simulink model "PV_microgrid"  (R2022b)
settings: Solver=FixedStepAuto  StartTime=0.0  StopTime=0.6  FixedStep=1e-6  RelTol=1e-3
model workspace (MAT data in the model file):
  C = 0.002
  D = 100
  GP = 1
  GQ = 1
  I1 = 100
  I2 = 50
  J = 3.5
  KQ = 0.06
  Kf = 120
  Kv = 577
  L = 2e-05
  LS = 0.003
  P1 = 0.2
  P2 = 6
  Pref = 500000
  Qref = 0
  Ts = 0.0001
  Ts_power = 1e-06
  Ug = 563.38264084
  fsw = 10000
  t0 = 0.5
  wn = 314.159265359
undefined symbols (not defined in the file): D1, Delta, DiscIntNeverNeededParam, Ion, Lithium, LL, LP, Ts_Power
libraries: spsSeriesRLCBranchLib x9, spsFirstOrderFilterLib x7, slpidlib x5, spsMeanLib x5, spsabctodq0Lib x4, spsStairGeneratorLib x4, spsThreePhaseVIMeasurementLib x3, spsThreePhaseTransformerTwoWindingsLib x2, spsThreePhaseParallelRLCLoadLib x2, spsThreePhasePISectionLineLib x2, spsBoostConverterLib x2, spsPowerPositiveSequenceLib x2
(part 2 of 2)

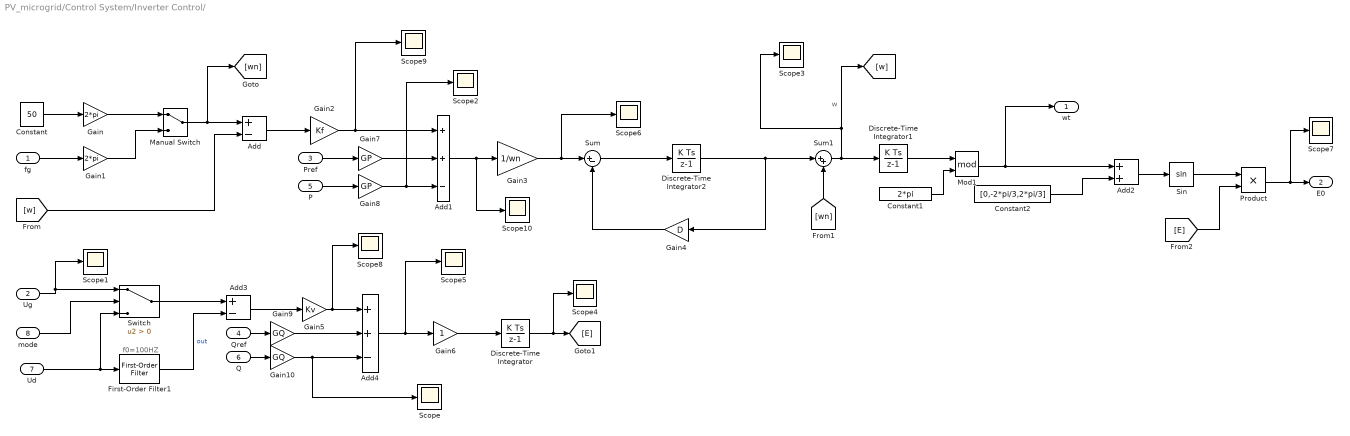
== system PV_microgrid/Control System/Inverter Control/   ==
  note: f0=100HZ
  note: w
  fg : Inport
  Ug : Inport  Port=2
  Pref : Inport  Port=3
  Qref : Inport  Port=4
  P : Inport  Port=5
  Q : Inport  Port=6
  Ud : Inport  Port=7
  mode : Inport  Port=8
  Add : Sum  Inputs=+-
  Add1 : Sum  Inputs=++-
  Add2 : Sum
  Add3 : Sum  Inputs=+-
  Add4 : Sum  Inputs=++-
  Constant : Constant  Value=50
  Constant1 : Constant  Value=2*pi
  Constant2 : Constant  Value=[0,-2*pi/3,2*pi/3]
  Discrete-Time Integrator : DiscreteIntegrator  gainval=KQ  SampleTime=1/fsw  ICPrevOutput=DiscIntNeverNeededParam  ICPrevScaledInput=DiscIntNeverNeededParam
  Discrete-Time Integrator1 : DiscreteIntegrator  SampleTime=1/fsw  ICPrevOutput=DiscIntNeverNeededParam  ICPrevScaledInput=DiscIntNeverNeededParam
  Discrete-Time Integrator2 : DiscreteIntegrator  gainval=1/J  SampleTime=1/fsw  ICPrevOutput=DiscIntNeverNeededParam  ICPrevScaledInput=DiscIntNeverNeededParam
  First-Order Filter1 : spsFirstOrderFilterLib/First-Order Filter  FilterType=Lowpass  Tc=10e-3  Ts=1/fsw  Initialize=on  Vac_Init=[0, 0, 10]  Vdc_Init=0  PlotResponse=off  FreqRange="[0,  200,  1]"
  Gain : Gain  Gain=2*pi
  Gain1 : Gain  Gain=2*pi
  Gain10 : Gain  Gain=GQ
  Gain2 : Gain  Gain=Kf
  Gain3 : Gain  Gain=1/wn
  Gain4 : Gain  Gain=D
  Gain5 : Gain  Gain=Kv
  Gain6 : Gain
  Gain7 : Gain  Gain=GP
  Gain8 : Gain  Gain=GP
  Gain9 : Gain  Gain=GQ
  Manual Switch : ManualSwitch
  Mod1 : Math  Operator=mod
  Product : Product
  Scope{,1..10} (11 alike) : Scope
  Sin : Trigonometry
  Sum : Sum  Inputs=|+-
  Sum1 : Sum  Inputs=|++
  Switch : Switch  Criteria=u2 > Threshold  SaturateOnIntegerOverflow=off  InputSameDT=off
  wt : Outport
  E0 : Outport  Port=2
  wires:
  Ug/1 -> Switch/1, Scope1/1
  Gain3/1 -> Scope6/1, Sum/1
  Gain2/1 -> Scope9/1, Add1/1
  Product/1 -> Scope7/1, E0/1
  Add/1 -> Gain2/1
  [E] -> Product/2
  Add4/1 -> Scope5/1, Gain6/1
  Mod1/1 -> wt/1, Add2/1
  Sum1/1 -> Discrete-Time Integrator1/1, Scope3/1, [w]
  fg/1 -> Gain1/1
  Constant2/1 -> Add2/2
  First-Order Filter1/1 -> Add3/2  "out"
  Ud/1 -> Switch/3, First-Order Filter1/1
  Constant/1 -> Gain/1
  Sin/1 -> Product/1
  Add2/1 -> Sin/1
  Gain4/1 -> Sum/2
  P/1 -> Gain8/1
  Gain/1 -> Manual Switch/1
  Gain1/1 -> Manual Switch/2
  Discrete-Time Integrator2/1 -> Gain4/1, Sum1/1
  Constant1/1 -> Mod1/2
  Gain5/1 -> Scope8/1, Add4/1
  Q/1 -> Gain10/1
  Manual Switch/1 -> [wn], Add/1
  Pref/1 -> Gain7/1
  Add1/1 -> Scope10/1, Gain3/1
  Add3/1 -> Gain5/1
  Gain6/1 -> Discrete-Time Integrator/1
  Qref/1 -> Gain9/1
  [wn] -> Sum1/2
  Sum/1 -> Discrete-Time Integrator2/1
  Discrete-Time Integrator/1 -> Scope4/1, [E]
  Discrete-Time Integrator1/1 -> Mod1/1
  [w] -> Add/2
  Gain7/1 -> Add1/2
  Gain8/1 -> Scope2/1, Add1/3
  Gain9/1 -> Add4/2
  Gain10/1 -> Scope/1, Add4/3
  Switch/1 -> Add3/1
  mode/1 -> Switch/2

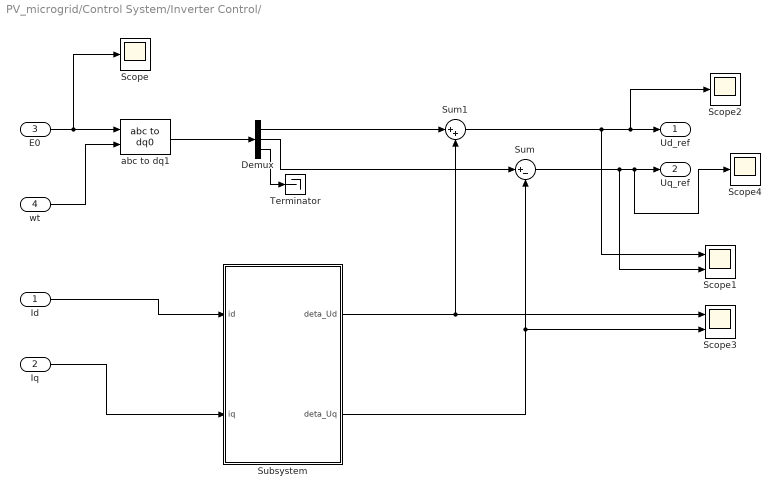
== system PV_microgrid/Control System/Inverter Control/    ==
  Id : Inport
  Iq : Inport  Port=2
  E0 : Inport  Description=Cont  Port=3
  wt : Inport  Port=4
  Demux : Demux  Outputs=3
  Scope : Scope
  Scope1 : Scope  NumInputPorts=2
  Scope2 : Scope
  Scope3 : Scope  NumInputPorts=2
  Scope4 : Scope
  Subsystem : Subsystem
  Sum : Sum  Inputs=|+-
  Sum1 : Sum  Inputs=|++
  Terminator : Terminator
  abc to dq1 : spsabctodq0Lib/abc to dq0  Alignment=90 degrees behind phase A axis
  Ud_ref : Outport
  Uq_ref : Outport  Port=2
  wires:
  Demux/1 -> Sum1/1
  E0/1 -> Scope/1, abc to dq1/1
  Id/1 -> Subsystem/1(id)
  abc to dq1/1 -> Demux/1
  Subsystem/2(deta_Uq) -> Scope3/2, Sum/2
  Sum1/1 -> Scope2/1, Ud_ref/1, Scope1/1
  wt/1 -> abc to dq1/2
  Demux/2 -> Sum/1
  Subsystem/1(deta_Ud) -> Sum1/2, Scope3/1
  Iq/1 -> Subsystem/2(iq)
  Sum/1 -> Scope4/1, Uq_ref/1, Scope1/2
  Demux/3 -> Terminator/1

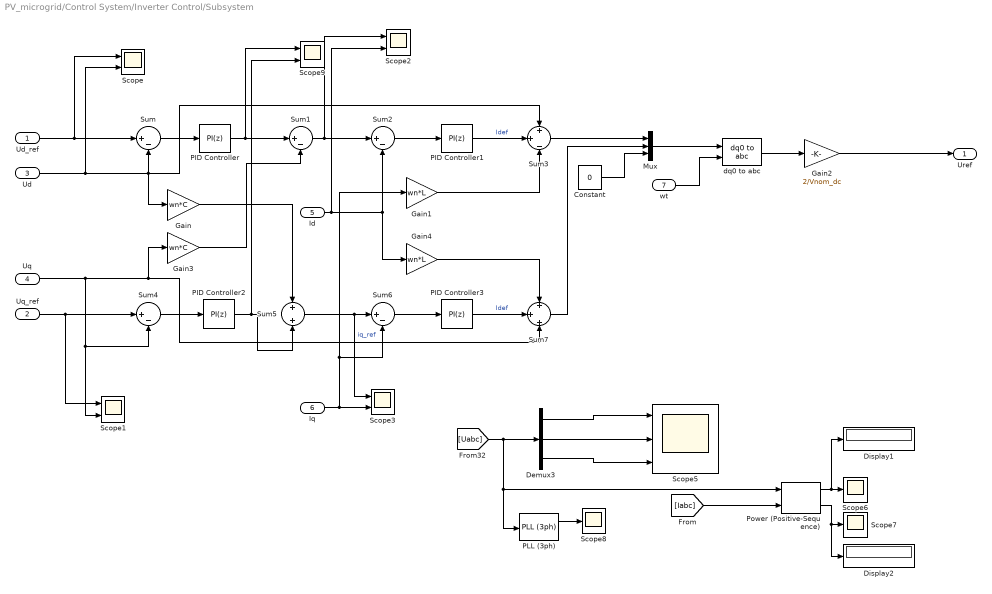
== system PV_microgrid/Control System/Inverter Control/Subsystem ==
  Ud_ref : Inport
  Uq_ref : Inport  Port=2
  Ud : Inport  Port=3
  Uq : Inport  Port=4
  Id : Inport  Port=5
  Iq : Inport  Port=6
  wt : Inport  Port=7
  Constant : Constant  Value=0
  Demux3 : Demux  Outputs=3
  Display1 : Display
  Display2 : Display
  Gain : Gain  Gain=wn*C
  Gain1 : Gain  Gain=wn*L
  Gain2 : Gain  Gain=2/Vnom_dc
  Gain3 : Gain  Gain=wn*C
  Gain4 : Gain  Gain=wn*L
  Mux : Mux  Inputs=3
  PID Controller : slpidlib/PID Controller  Controller=PI  Form=Parallel  TimeDomain=Discrete-time  UseExternalTs=off  SampleTime=-1  IntegratorMethod=Forward Euler  FilterMethod=Forward Euler  ControllerParametersSource=internal  P=P1  I=I1  UseKiTs=off  D=0  N=100  UseFilter=on  TunerSelectOption=Transfer Function Based (PID Tuner App)  InitialConditionSource=internal  InitialConditionForIntegrator=0  InitialConditionForFilter=0  DifferentiatorICPrevScaledInput=0  ExternalReset=none  TrackingMode=off  Kt=1  LimitOutput=off  SatLimitsSource=internal  UpperSaturationLimit=LP  LowerSaturationLimit=LL  LinearizeAsGain=on  AntiWindupMode=none  Kb=1  LimitIntegrator=off  UpperIntegratorSaturationLimit=inf  LowerIntegratorSaturationLimit=-inf  POutMin=[]  POutMax=[]  IOutMin=[]  IOutMax=[]  DOutMin=[]  DOutMax=[]  NOutMin=[]  NOutMax=[]  SumOutMin=[]  SumOutMax=[]  SaturationOutMin=[]  SaturationOutMax=[]  PParamMin=[]  PParamMax=[]  IParamMin=[]  IParamMax=[]  DParamMin=[]  DParamMax=[]  NParamMin=[]  NParamMax=[]  KbParamMin=[]  KbParamMax=[]  KtParamMin=[]  KtParamMax=[]  KbOutMin=[]  KbOutMax=[]  KtOutMin=[]  KtOutMax=[]  IntegratorOutMin=[]  IntegratorOutMax=[]  FilterOutMin=[]  FilterOutMax=[]  SumI1OutMin=[]  SumI1OutMax=[]  SumI2OutMin=[]  SumI2OutMax=[]  SumI3OutMin=[]  SumI3OutMax=[]  SumI4OutMin=[]  SumI4OutMax=[]  SumDOutMin=[]  SumDOutMax=[]  DifferentiatorOutMin=[]  DifferentiatorOutMax=[]  FilterDiffOutCoefMin=[]  FilterDiffOutCoefMax=[]  ReciprocalOutMin=[]  ReciprocalOutMax=[]  SumDenOutMin=[]  SumDenOutMax=[]  SumNumOutMin=[]  SumNumOutMax=[]  DivideOutMin=[]  DivideOutMax=[]  UdiffTsProdOutMin=[]  UdiffTsProdOutMax=[]  NTsProdOutMin=[]  NTsProdOutMax=[]  UintegralTsProdOutMin=[]  UintegralTsProdOutMax=[]  UngainTsProdOutMin=[]  UngainTsProdOutMax=[]  ClampingZeroOutDataTypeStr=Inherit: Inherit via back propagation  ClampingZeroOutMin=[]  ClampingZeroOutMax=[]  FilterDenConstantOutDataTypeStr=Inherit: Inherit via back propagation  FilterDenConstantOutMin=[]  FilterDenConstantOutMax=[]  PCopyOutDataTypeStr=Inherit: Inherit via back propagation  PCopyOutMin=[]  PCopyOutMax=[]  NCopyOutDataTypeStr=Inherit: Inherit via back propagation  NCopyOutMin=[]  NCopyOutMax=[]  IntegratorContinuousStateAttributes=''  IntegratorStateMustResolveToSignalObject=off  IntegratorRTWStateStorageClass=Auto  FilterContinuousStateAttributes=''  FilterStateMustResolveToSignalObject=off  FilterRTWStateStorageClass=Auto  ParallelPVariant=InternalParameters  IdealPVariant=Disabled  IVariant=InternalParameters  DVariant=Disabled  IntegratorVariant=Discrete  SatVariant=Disabled  AWVariant=Passthrough  PCopyVariant=Disabled  TRVariant=Disabled  FdbkBlocksVariant=Forward  IdealPFdbkVariant=Disabled  SatFdbkVariant=Disabled  DerivativeFilterVariant=Disabled  NVariant=Disabled  NCopyVariant=Disabled_SignalSpec  FilterICVariant=Disabled  IntegratorICVariant=InternalICs  ExternalResetVariant=Disabled  TRSumVariant=Passthrough  SumFdbkVariant=Disabled  SumVariant=Sum_PI  TsampFilterVariant=InternalTs  TsampNgainVariant=Passthrough  TsampIntegralVariant=Passthrough  ExternalSaturationOutDataTypeStr=Inherit: Same as second input
  PID Controller1 : slpidlib/PID Controller  Controller=PI  Form=Parallel  TimeDomain=Discrete-time  UseExternalTs=off  SampleTime=-1  IntegratorMethod=Forward Euler  FilterMethod=Forward Euler  ControllerParametersSource=internal  P=P2  I=I2  UseKiTs=off  D=0  N=100  UseFilter=on  TunerSelectOption=Transfer Function Based (PID Tuner App)  InitialConditionSource=internal  InitialConditionForIntegrator=0  InitialConditionForFilter=0  DifferentiatorICPrevScaledInput=0  ExternalReset=none  TrackingMode=off  Kt=1  LimitOutput=off  SatLimitsSource=internal  UpperSaturationLimit=inf  LowerSaturationLimit=-inf  LinearizeAsGain=on  AntiWindupMode=none  Kb=1  LimitIntegrator=off  UpperIntegratorSaturationLimit=inf  LowerIntegratorSaturationLimit=-inf  POutMin=[]  POutMax=[]  IOutMin=[]  IOutMax=[]  DOutMin=[]  DOutMax=[]  NOutMin=[]  NOutMax=[]  SumOutMin=[]  SumOutMax=[]  SaturationOutMin=[]  SaturationOutMax=[]  PParamMin=[]  PParamMax=[]  IParamMin=[]  IParamMax=[]  DParamMin=[]  DParamMax=[]  NParamMin=[]  NParamMax=[]  KbParamMin=[]  KbParamMax=[]  KtParamMin=[]  KtParamMax=[]  KbOutMin=[]  KbOutMax=[]  KtOutMin=[]  KtOutMax=[]  IntegratorOutMin=[]  IntegratorOutMax=[]  FilterOutMin=[]  FilterOutMax=[]  SumI1OutMin=[]  SumI1OutMax=[]  SumI2OutMin=[]  SumI2OutMax=[]  SumI3OutMin=[]  SumI3OutMax=[]  SumI4OutMin=[]  SumI4OutMax=[]  SumDOutMin=[]  SumDOutMax=[]  DifferentiatorOutMin=[]  DifferentiatorOutMax=[]  FilterDiffOutCoefMin=[]  FilterDiffOutCoefMax=[]  ReciprocalOutMin=[]  ReciprocalOutMax=[]  SumDenOutMin=[]  SumDenOutMax=[]  SumNumOutMin=[]  SumNumOutMax=[]  DivideOutMin=[]  DivideOutMax=[]  UdiffTsProdOutMin=[]  UdiffTsProdOutMax=[]  NTsProdOutMin=[]  NTsProdOutMax=[]  UintegralTsProdOutMin=[]  UintegralTsProdOutMax=[]  UngainTsProdOutMin=[]  UngainTsProdOutMax=[]  ClampingZeroOutDataTypeStr=Inherit: Inherit via back propagation  ClampingZeroOutMin=[]  ClampingZeroOutMax=[]  FilterDenConstantOutDataTypeStr=Inherit: Inherit via back propagation  FilterDenConstantOutMin=[]  FilterDenConstantOutMax=[]  PCopyOutDataTypeStr=Inherit: Inherit via back propagation  PCopyOutMin=[]  PCopyOutMax=[]  NCopyOutDataTypeStr=Inherit: Inherit via back propagation  NCopyOutMin=[]  NCopyOutMax=[]  IntegratorContinuousStateAttributes=''  IntegratorStateMustResolveToSignalObject=off  IntegratorRTWStateStorageClass=Auto  FilterContinuousStateAttributes=''  FilterStateMustResolveToSignalObject=off  FilterRTWStateStorageClass=Auto  ParallelPVariant=InternalParameters  IdealPVariant=Disabled  IVariant=InternalParameters  DVariant=Disabled  IntegratorVariant=Discrete  SatVariant=Disabled  AWVariant=Passthrough  PCopyVariant=Disabled  TRVariant=Disabled  FdbkBlocksVariant=Forward  IdealPFdbkVariant=Disabled  SatFdbkVariant=Disabled  DerivativeFilterVariant=Disabled  NVariant=Disabled  NCopyVariant=Disabled_SignalSpec  FilterICVariant=Disabled  IntegratorICVariant=InternalICs  ExternalResetVariant=Disabled  TRSumVariant=Passthrough  SumFdbkVariant=Disabled  SumVariant=Sum_PI  TsampFilterVariant=InternalTs  TsampNgainVariant=Passthrough  TsampIntegralVariant=Passthrough  ExternalSaturationOutDataTypeStr=Inherit: Same as second input
  PID Controller2 : slpidlib/PID Controller  Controller=PI  Form=Parallel  TimeDomain=Discrete-time  UseExternalTs=off  SampleTime=-1  IntegratorMethod=Forward Euler  FilterMethod=Forward Euler  ControllerParametersSource=internal  P=P1  I=I1  UseKiTs=off  D=0  N=100  UseFilter=on  TunerSelectOption=Transfer Function Based (PID Tuner App)  InitialConditionSource=internal  InitialConditionForIntegrator=0  InitialConditionForFilter=0  DifferentiatorICPrevScaledInput=0  ExternalReset=none  TrackingMode=off  Kt=1  LimitOutput=off  SatLimitsSource=internal  UpperSaturationLimit=LP  LowerSaturationLimit=LL  LinearizeAsGain=on  AntiWindupMode=none  Kb=1  LimitIntegrator=off  UpperIntegratorSaturationLimit=inf  LowerIntegratorSaturationLimit=-inf  POutMin=[]  POutMax=[]  IOutMin=[]  IOutMax=[]  DOutMin=[]  DOutMax=[]  NOutMin=[]  NOutMax=[]  SumOutMin=[]  SumOutMax=[]  SaturationOutMin=[]  SaturationOutMax=[]  PParamMin=[]  PParamMax=[]  IParamMin=[]  IParamMax=[]  DParamMin=[]  DParamMax=[]  NParamMin=[]  NParamMax=[]  KbParamMin=[]  KbParamMax=[]  KtParamMin=[]  KtParamMax=[]  KbOutMin=[]  KbOutMax=[]  KtOutMin=[]  KtOutMax=[]  IntegratorOutMin=[]  IntegratorOutMax=[]  FilterOutMin=[]  FilterOutMax=[]  SumI1OutMin=[]  SumI1OutMax=[]  SumI2OutMin=[]  SumI2OutMax=[]  SumI3OutMin=[]  SumI3OutMax=[]  SumI4OutMin=[]  SumI4OutMax=[]  SumDOutMin=[]  SumDOutMax=[]  DifferentiatorOutMin=[]  DifferentiatorOutMax=[]  FilterDiffOutCoefMin=[]  FilterDiffOutCoefMax=[]  ReciprocalOutMin=[]  ReciprocalOutMax=[]  SumDenOutMin=[]  SumDenOutMax=[]  SumNumOutMin=[]  SumNumOutMax=[]  DivideOutMin=[]  DivideOutMax=[]  UdiffTsProdOutMin=[]  UdiffTsProdOutMax=[]  NTsProdOutMin=[]  NTsProdOutMax=[]  UintegralTsProdOutMin=[]  UintegralTsProdOutMax=[]  UngainTsProdOutMin=[]  UngainTsProdOutMax=[]  ClampingZeroOutDataTypeStr=Inherit: Inherit via back propagation  ClampingZeroOutMin=[]  ClampingZeroOutMax=[]  FilterDenConstantOutDataTypeStr=Inherit: Inherit via back propagation  FilterDenConstantOutMin=[]  FilterDenConstantOutMax=[]  PCopyOutDataTypeStr=Inherit: Inherit via back propagation  PCopyOutMin=[]  PCopyOutMax=[]  NCopyOutDataTypeStr=Inherit: Inherit via back propagation  NCopyOutMin=[]  NCopyOutMax=[]  IntegratorContinuousStateAttributes=''  IntegratorStateMustResolveToSignalObject=off  IntegratorRTWStateStorageClass=Auto  FilterContinuousStateAttributes=''  FilterStateMustResolveToSignalObject=off  FilterRTWStateStorageClass=Auto  ParallelPVariant=InternalParameters  IdealPVariant=Disabled  IVariant=InternalParameters  DVariant=Disabled  IntegratorVariant=Discrete  SatVariant=Disabled  AWVariant=Passthrough  PCopyVariant=Disabled  TRVariant=Disabled  FdbkBlocksVariant=Forward  IdealPFdbkVariant=Disabled  SatFdbkVariant=Disabled  DerivativeFilterVariant=Disabled  NVariant=Disabled  NCopyVariant=Disabled_SignalSpec  FilterICVariant=Disabled  IntegratorICVariant=InternalICs  ExternalResetVariant=Disabled  TRSumVariant=Passthrough  SumFdbkVariant=Disabled  SumVariant=Sum_PI  TsampFilterVariant=InternalTs  TsampNgainVariant=Passthrough  TsampIntegralVariant=Passthrough  ExternalSaturationOutDataTypeStr=Inherit: Same as second input
  PID Controller3 : slpidlib/PID Controller  Controller=PI  Form=Parallel  TimeDomain=Discrete-time  UseExternalTs=off  SampleTime=-1  IntegratorMethod=Forward Euler  FilterMethod=Forward Euler  ControllerParametersSource=internal  P=P2  I=I2  UseKiTs=off  D=0  N=100  UseFilter=on  TunerSelectOption=Transfer Function Based (PID Tuner App)  InitialConditionSource=internal  InitialConditionForIntegrator=0  InitialConditionForFilter=0  DifferentiatorICPrevScaledInput=0  ExternalReset=none  TrackingMode=off  Kt=1  LimitOutput=off  SatLimitsSource=internal  UpperSaturationLimit=inf  LowerSaturationLimit=-inf  LinearizeAsGain=on  AntiWindupMode=none  Kb=1  LimitIntegrator=off  UpperIntegratorSaturationLimit=inf  LowerIntegratorSaturationLimit=-inf  POutMin=[]  POutMax=[]  IOutMin=[]  IOutMax=[]  DOutMin=[]  DOutMax=[]  NOutMin=[]  NOutMax=[]  SumOutMin=[]  SumOutMax=[]  SaturationOutMin=[]  SaturationOutMax=[]  PParamMin=[]  PParamMax=[]  IParamMin=[]  IParamMax=[]  DParamMin=[]  DParamMax=[]  NParamMin=[]  NParamMax=[]  KbParamMin=[]  KbParamMax=[]  KtParamMin=[]  KtParamMax=[]  KbOutMin=[]  KbOutMax=[]  KtOutMin=[]  KtOutMax=[]  IntegratorOutMin=[]  IntegratorOutMax=[]  FilterOutMin=[]  FilterOutMax=[]  SumI1OutMin=[]  SumI1OutMax=[]  SumI2OutMin=[]  SumI2OutMax=[]  SumI3OutMin=[]  SumI3OutMax=[]  SumI4OutMin=[]  SumI4OutMax=[]  SumDOutMin=[]  SumDOutMax=[]  DifferentiatorOutMin=[]  DifferentiatorOutMax=[]  FilterDiffOutCoefMin=[]  FilterDiffOutCoefMax=[]  ReciprocalOutMin=[]  ReciprocalOutMax=[]  SumDenOutMin=[]  SumDenOutMax=[]  SumNumOutMin=[]  SumNumOutMax=[]  DivideOutMin=[]  DivideOutMax=[]  UdiffTsProdOutMin=[]  UdiffTsProdOutMax=[]  NTsProdOutMin=[]  NTsProdOutMax=[]  UintegralTsProdOutMin=[]  UintegralTsProdOutMax=[]  UngainTsProdOutMin=[]  UngainTsProdOutMax=[]  ClampingZeroOutDataTypeStr=Inherit: Inherit via back propagation  ClampingZeroOutMin=[]  ClampingZeroOutMax=[]  FilterDenConstantOutDataTypeStr=Inherit: Inherit via back propagation  FilterDenConstantOutMin=[]  FilterDenConstantOutMax=[]  PCopyOutDataTypeStr=Inherit: Inherit via back propagation  PCopyOutMin=[]  PCopyOutMax=[]  NCopyOutDataTypeStr=Inherit: Inherit via back propagation  NCopyOutMin=[]  NCopyOutMax=[]  IntegratorContinuousStateAttributes=''  IntegratorStateMustResolveToSignalObject=off  IntegratorRTWStateStorageClass=Auto  FilterContinuousStateAttributes=''  FilterStateMustResolveToSignalObject=off  FilterRTWStateStorageClass=Auto  ParallelPVariant=InternalParameters  IdealPVariant=Disabled  IVariant=InternalParameters  DVariant=Disabled  IntegratorVariant=Discrete  SatVariant=Disabled  AWVariant=Passthrough  PCopyVariant=Disabled  TRVariant=Disabled  FdbkBlocksVariant=Forward  IdealPFdbkVariant=Disabled  SatFdbkVariant=Disabled  DerivativeFilterVariant=Disabled  NVariant=Disabled  NCopyVariant=Disabled_SignalSpec  FilterICVariant=Disabled  IntegratorICVariant=InternalICs  ExternalResetVariant=Disabled  TRSumVariant=Passthrough  SumFdbkVariant=Disabled  SumVariant=Sum_PI  TsampFilterVariant=InternalTs  TsampNgainVariant=Passthrough  TsampIntegralVariant=Passthrough  ExternalSaturationOutDataTypeStr=Inherit: Same as second input
  PLL (3ph) : spsPLL3phLib/PLL (3ph)  Fmin=45  Par_Init=[0, 50]  ParK=[180, 3200, 1]  TcD=1e-4  MaxRateChangeFreq=12  FilterCutOffFreq=25  Ts=1/fsw  AGC=on
  Power (Positive-Sequence) : spsPowerPositiveSequenceLib/Power (Positive-Sequence)  Freq=50  Vinit=[0, 0]  Iinit=[0, 0]  Ts=1/fsw
      settings: LibrarySourceBlock=|
      | sps_lib/Sensors and Measurements/Power
      | (Positive-Sequence)
  Scope{,1..3,9} (5 alike) : Scope  NumInputPorts=2
  Scope5 : Scope  NumInputPorts=3
  Scope6 : Scope
  Scope7 : Scope
  Scope8 : Scope
  Sum{,1..2,4,6} (5 alike) : Sum  Inputs=|+-
  Sum3 : Sum  Inputs=+|+|-
  Sum5 : Sum  Inputs=+|+
  Sum7 : Sum  Inputs=+|+|+
  dq0 to abc : spsdq0toabcLib/dq0 to abc  Alignment=90 degrees behind phase A axis
  Uref : Outport
  wires:
  Constant/1 -> Mux/3
  PID Controller2/1 -> Scope9/2, Sum5/2
  wt/1 -> dq0 to abc/2
  Mux/1 -> dq0 to abc/1
  Ud_ref/1 -> Scope/1, Sum/1
  Iq/1 -> Gain1/1, Sum6/2, Scope3/2
  Uq/1 -> Sum4/2, Scope1/2, Sum7/3, Gain3/1
  Sum3/1 -> Mux/1
  Sum5/1 -> Scope3/1, Sum6/1  "iq_ref"
  Sum2/1 -> PID Controller1/1
  Sum/1 -> PID Controller/1
  Sum7/1 -> Mux/2
  PID Controller1/1 -> Sum3/2  "Idef"
  Gain/1 -> Sum5/1
  Uq_ref/1 -> Scope1/1, Sum4/1
  Ud/1 -> Scope/2, Sum/2, Sum3/1, Gain/1
  Sum6/1 -> PID Controller3/1
  Sum4/1 -> PID Controller2/1
  Id/1 -> Gain4/1, Sum2/2, Scope2/2
  PID Controller3/1 -> Sum7/2  "Idef"
  Gain2/1 -> Uref/1
  dq0 to abc/1 -> Gain2/1
  Gain3/1 -> Sum1/2
  Sum1/1 -> Scope2/1, Sum2/1
  Gain1/1 -> Sum3/3
  Gain4/1 -> Sum7/1
  PLL (3ph)/1 -> Scope8/1
  [Iabc] -> Power (Positive-Sequence)/2
  Demux3/1 -> Scope5/1
  Demux3/2 -> Scope5/2
  Power (Positive-Sequence)/1 -> Display1/1, Scope6/1
  [Uabc] -> PLL (3ph)/1, Power (Positive-Sequence)/1, Demux3/1
  Power (Positive-Sequence)/2 -> Display2/1, Scope7/1
  Demux3/3 -> Scope5/3
  PID Controller/1 -> Scope9/1, Sum1/1

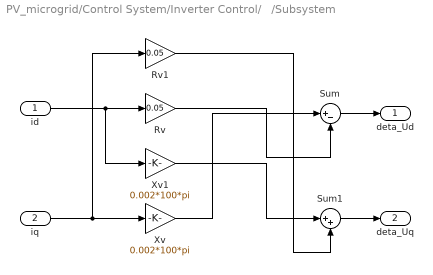
== system PV_microgrid/Control System/Inverter Control/   /Subsystem ==
  id : Inport
  iq : Inport  Port=2
  Rv : Gain  Gain=0.05
  Rv1 : Gain  Gain=0.05
  Sum : Sum  Inputs=|+-
  Sum1 : Sum  Inputs=|++
  Xv : Gain  Gain=0.002*100*pi
  Xv1 : Gain  Gain=0.002*100*pi
  deta_Ud : Outport
  deta_Uq : Outport  Port=2
  wires:
  Sum/1 -> deta_Ud/1
  Sum1/1 -> deta_Uq/1
  id/1 -> Xv1/1, Rv/1
  Rv/1 -> Sum/2
  iq/1 -> Rv1/1, Xv/1
  Xv/1 -> Sum/1
  Xv1/1 -> Sum1/1
  Rv1/1 -> Sum1/2

== matlab function PV_microgrid/Control System/MPPT Controller 2/MPPT Control 1  ==
  settings: updateMethod=DISCRETE  sampleTime=Ts
  data: V input =V; I input; D output; Dmax parameter; Dmin parameter; deltaD parameter; Dinit parameter
function D  = PandO(V, I, Dmax, Dmin, deltaD, Dinit)

% MPPT controller based on the Perturb & Observe algorithm.

% D output = Duty cycle of the boost converter (value between 0 and 1)
% V input = PV array terminal voltage (V)
% I input = PV array current (A)
% D = 1 - Vinput/Voutput (increasing D decrease Vin)

persistent Vold Pold Dold;
%
if isempty(Vold)
    Vold=0;
    Pold=0;
    Dold=Dinit;
end
P= V*I;
dV= V - Vold;
dP= P - Pold;
%
% if dP ~= 0
    if dP < 0
        if dV < 0
            D = Dold - deltaD;
        else
            D = Dold + deltaD;
        end
    else
        if dV < 0
            D = Dold + deltaD;
        else
            D = Dold - deltaD;
        end    
    end
% else
%     D=Dold;
% end
%
if D >= Dmax || D<= Dmin
    D=Dold;
end
%
Dold=D;
Vold=V;
Pold=P;

== matlab function PV_microgrid/Control System/MPPT Controller 1/MPPT Control 1  ==
  settings: updateMethod=DISCRETE  sampleTime=Ts
  data: V input =V; I input; D output; Dmax parameter; Dmin parameter; deltaD parameter; Dinit parameter
function D  = PandO(V, I, Dmax, Dmin, deltaD, Dinit)

% MPPT controller based on the Perturb & Observe algorithm.

% D output = Duty cycle of the boost converter (value between 0 and 1)
% V input = PV array terminal voltage (V)
% I input = PV array current (A)
% D = 1 - Vinput/Voutput (increasing D decrease Vin)

persistent Vold Pold Dold;
%
if isempty(Vold)
    Vold=0;
    Pold=0;
    Dold=Dinit;
end
P= V*I;
dV= V - Vold;
dP= P - Pold;
%
% if dP ~= 0
    if dP < 0
        if dV < 0
            D = Dold - deltaD;
        else
            D = Dold + deltaD;
        end
    else
        if dV < 0
            D = Dold + deltaD;
        else
            D = Dold - deltaD;
        end    
    end
% else
%     D=Dold;
% end
%
if D >= Dmax || D<= Dmin
    D=Dold;
end
%
Dold=D;
Vold=V;
Pold=P;
